simulink model "spring_mass_dumper_system"  (R2023b)
settings: Solver=VariableStepAuto  StartTime=0.0  StopTime=10.0  RelTol=1e-3
settings Model: Creator=yowov  LastModifiedBy=yowov

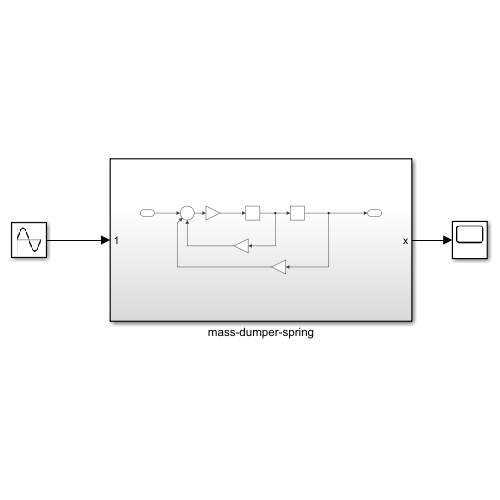
[thumbnail: Simulink's stored preview of the top-level diagram]
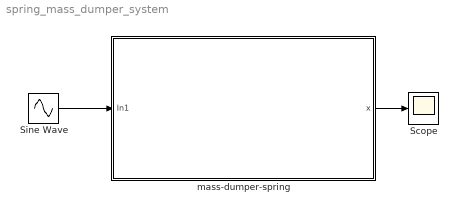
== system spring_mass_dumper_system ==
  Scope : Scope
  Sine Wave : Sin  Amplitude=2  Frequency=2  SampleTime=0
  mass-dumper-spring : Subsystem
  wires:
  Sine Wave/1 -> mass-dumper-spring/1(In1)
  mass-dumper-spring/1(x) -> Scope/1

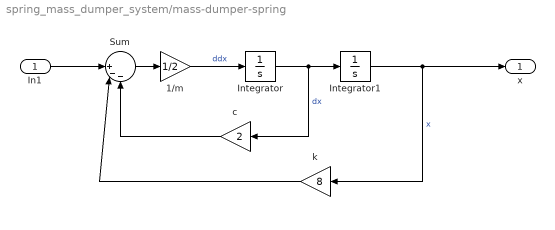
== system spring_mass_dumper_system/mass-dumper-spring ==
  In1 : Inport
  1/m : Gain  Gain=1/2
  Integrator : Integrator  InitialCondition=2
  Integrator1 : Integrator  InitialCondition=1
  Sum : Sum  Inputs=||+--
  c : Gain  Gain=2
  k : Gain  Gain=8
  x : Outport
  wires:
  Integrator/1 -> c/1, Integrator1/1  "dx"
  Integrator1/1 -> x/1, k/1  "x"
  c/1 -> Sum/3
  In1/1 -> Sum/1
  k/1 -> Sum/2
  1/m/1 -> Integrator/1  "ddx"
  Sum/1 -> 1/m/1
